simulink model "RB_KAIROS_impControl_compensation"  (R2020b)
settings: Solver=ode4  StartTime=0.0  StopTime=t_end  FixedStep=Ts  RelTol=1e-3
values from neighbouring files (symbols this model uses):
  am = 0.3    [RB_KAIROS_ImpControl_OpSpace_quat_2020b_safety_main.m]
  am_r = 0.3    [RB_KAIROS_ImpControl_OpSpace_quat_2020b_safety_main.m]
  Kc = diag(50*ones(6,1))    [RB_KAIROS_ImpControl_OpSpace_quat_2020b_safety_main.m]
  Kp = 2*[400;400;400;400;0;0;0]    [RB_KAIROS_ImpControl_OpSpace_quat_2020b_safety_main.m]
  Kv = [1000;1000;1000;[300;300;300;300;300;300;300]]    [RB_KAIROS_ImpControl_OpSpace_quat_2020b_safety_main.m]
  model_sample_time = 0.001    [RB_KAIROS_ImpControl_OpSpace_quat_2020b_safety_main.m]
  q_dot_0 = zeros(10,1)    [RB_KAIROS_ImpControl_OpSpace_quat_2020b_safety_main.m]
  T_i = K    [RB_KAIROS_ImpControl_OpSpace_quat_2020b_safety_main.m]
  tau_ext = [0 0 0 0 0 0 0 0 0 0 0]    [RB_KAIROS_ImpControl_OpSpace_quat_2020b_safety_main.m]
  v_SMU = 10    [RB_KAIROS_ImpControl_OpSpace_quat_2020b_safety_main.m]
  vm = 0.5    [RB_KAIROS_ImpControl_OpSpace_quat_2020b_safety_main.m]
  vm_r = 0.5    [RB_KAIROS_ImpControl_OpSpace_quat_2020b_safety_main.m]
undefined symbols (not defined in the file or in its folder): DiscIntNeverNeededParam, magnitude, q_0, T_f
libraries: simulink x4, utils x4, transformations_lib x3
(part 18 of 18)

== matlab function RB_KAIROS_impControl_compensation/Trajectory Generator/move2pose/MATLAB Function ==
  data: in input; reset input; out output
function out = fcn(in,reset)
%%% This is kind of a Memory block for one boolean.
% output is equal input as long as input is not zero.
% If input becomes zero, output STAYS zero, till reset is triggered.


persistent memory 
if isempty(memory)
    memory = 0;       %remembers the state
end

out = in;

if in == 0
    memory = 1;
end

if memory == 1
    out = 0;
    if reset>0
        memory = 0;
    end
end

end

== matlab function RB_KAIROS_impControl_compensation/Trajectory Generator/Subsystem1/Angle Axis Via Quaternions/r2q ==
  data: R input; q output
function q =r2q(R)
%#codegen
q=zeros(1,4);
if ~(all(size(R)==[3,3]))
    error('Bad input dimensions. Input must be 3x3');
end

% Ne dela za specialne kote, ko je s=0 ali v=0
% s=0.5*sqrt(R(1,1)+R(2,2)+R(3,3)+1);
% v=[R(3,2)-R(2,3),R(1,3)-R(3,1),R(2,1)-R(1,2)]'/4/s;
%
% q=quaternion([s v']);

qsx=trace(R)+1;
if qsx>=0
    qs = sqrt(qsx)/2.0;
else
    qs=0;
end
kx = R(3,2) - R(2,3);	% Oz - Ay
ky = R(1,3) - R(3,1);	% Ax - Nz
kz = R(2,1) - R(1,2);	% Ny - Ox

if (R(1,1) >= R(2,2)) && (R(1,1) >= R(3,3))
    kx1 = R(1,1) - R(2,2) - R(3,3) + 1;	% Nx - Oy - Az + 1
    ky1 = R(2,1) + R(1,2);			% Ny + Ox
    kz1 = R(3,1) + R(1,3);			% Nz + Ax
    add = (kx >= 0);
elseif (R(2,2) >= R(3,3))
    kx1 = R(2,1) + R(1,2);			% Ny + Ox
    ky1 = R(2,2) - R(1,1) - R(3,3) + 1;	% Oy - Nx - Az + 1
    kz1 = R(3,2) + R(2,3);			% Oz + Ay
    add = (ky >= 0);
else
    kx1 = R(3,1) + R(1,3);			% Nz + Ax
    ky1 = R(3,2) + R(2,3);			% Oz + Ay
    kz1 = R(3,3) - R(1,1) - R(2,2) + 1;	% Az - Nx - Oy + 1
    add = (kz >= 0);
end

if add
    kx = kx + kx1;
    ky = ky + ky1;
    kz = kz + kz1;
else
    kx = kx - kx1;
    ky = ky - ky1;
    kz = kz - kz1;
end
nm = norm([kx ky kz]);
if nm == 0
    q = [1 0 0 0];
else
    ss=1-qs^2;
    if ss<0
        s=0;
    else
        s = sqrt(ss) / nm;
    end
    qv = s*[kx ky kz];
    
    q = [qs qv];
end
